simulink library "csu_esf_est_switch_frame_mtv_lib"  (R2014b)
settings: Solver=ode45  StartTime=0.0  StopTime=10.0  RelTol=1e-3
values from neighbouring files (symbols this model uses):
  kfl_accel_init = [0 0 0]'    [csc_kfl_kalman_filter_mtv_init.m]
  kfl_convergence_init = 2    [csc_kfl_kalman_filter_mtv_init.m]
  kfl_integrating_init = 1    [csc_kfl_kalman_filter_mtv_init.m]
  kfl_landed_init = 0    [csc_kfl_kalman_filter_mtv_init.m]
  kfl_quat_init = kfl_ic.quat_eci_to_body    [csc_est_state_estimation_test.m]    (also in csc_kfl_kalman_filter_mtv_init.m = [0 0 0 1]')
  kfl_rate_init = [ 0 0 0]'    [csc_kfl_kalman_filter_mtv_init.m]
  kfl_state_init = [ kfl_position_init ; kfl_velocity_init ; kfl_acc_bias_init ;  kfl_gibbs_init ;  kfl_gyro_bias_init]    [csc_est_state_estimation_test.m]
undefined symbols (not defined in the file or in its folder): ekf_covariance_init, elk_body_base_to_origin, elk_launchstand_height
libraries: simulink x2, util_info_lib x1, util_event_lib x1, util_fsw_frame_rotation_lib x1
settings Model: Creator=escrane  LastModifiedBy=mstewart

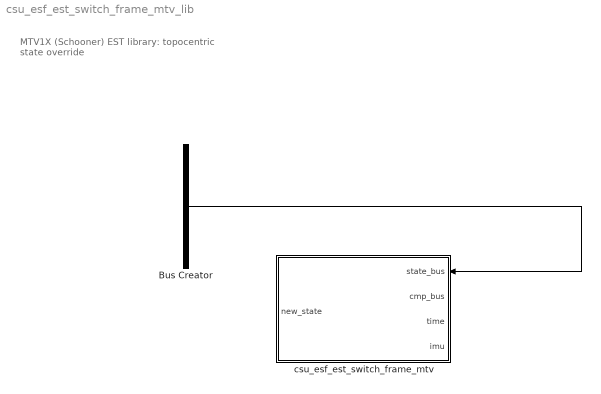
== system csu_esf_est_switch_frame_mtv_lib ==
  note: MTV1X (Schooner) EST library:
      | topocentric state override
  Bus Creator : BusCreator  Inputs=5
  csu_esf_est_switch_frame_mtv : Subsystem
  wires:
  Bus Creator/1 -> csu_esf_est_switch_frame_mtv/1(state_bus)
  ? -> Bus Creator/1  "x"
  ? -> Bus Creator/2  "accel"
  ? -> Bus Creator/3  "rate"
  ? -> Bus Creator/4  "q"
  ? -> Bus Creator/5  "P"

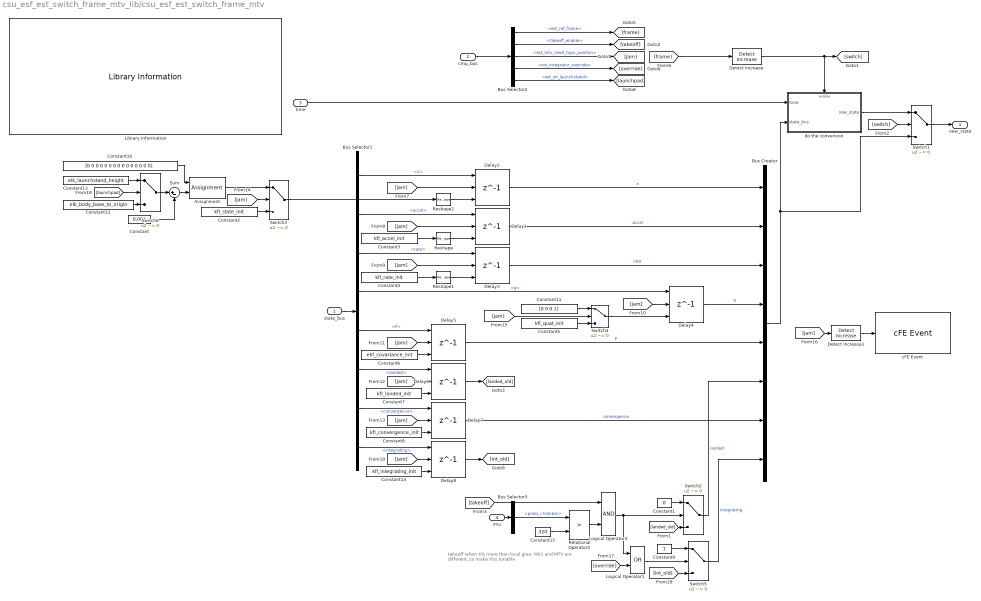
== system csu_esf_est_switch_frame_mtv_lib/csu_esf_est_switch_frame_mtv ==
  note: takeoff when X% more than local grav:
      | MX1 and MTV are different, so make this tunable
  state_bus : Inport
  cmp_bus : Inport  Port=2
  time : Inport  Port=3
  imu : Inport  Port=4
  Assignment : Assignment  DiagnosticForDimensions=Warning  Indices=3
  Bus Creator : BusCreator  Inputs=8
  Bus Selector1 : BusSelector  OutputSignals=x,accel,rate,q,P,landed,convergence,integrating
  Bus Selector2 : BusSelector  OutputSignals=est_ref_frame,takeoff_enable,est_mtv_reset_topo_position,est_integrator_override,est_on_launchstand
  Bus Selector3 : BusSelector  OutputSignals=press_chamber
  Constant : Constant  Value=0.001
  Constant1 : Constant  Value=0
  Constant10 : Constant  Value=[0 0 0 0 0 0 0 0 0 0 0 0 0 0 0]
  Constant11 : Constant  Value=[0 0 0 1]
  Constant12 : Constant  Value=elk_body_base_to_origin  VectorParams1D=off
  Constant13 : Constant  Value=elk_launchstand_height  VectorParams1D=off
  Constant14 : Constant  Value=kfl_integrating_init
  Constant15 : Constant  Value=320
  Constant2 : Constant  Value=kfl_state_init
  Constant3 : Constant  Value=kfl_accel_init
  Constant4 : Constant  Value=kfl_rate_init
  Constant5 : Constant  Value=kfl_quat_init
  Constant6 : Constant  Value=ekf_covariance_init
  Constant7 : Constant  Value=kfl_landed_init
  Constant8 : Constant  Value=kfl_convergence_init
  Constant9 : Constant
  Delay{1..8} (8 alike) : Delay  DelayLength=1  InitialConditionSource=Input port  ExternalReset=Rising
      settings: InputPortMap=u0,r5,p4
  Detect Increase : simulink/Logic and Bit Operations/Detect Increase  vinit=1  InputProcessing=Inherited  OutDataTypeStr=boolean
  Detect Increase1 : simulink/Logic and Bit Operations/Detect Increase  vinit=0  InputProcessing=Inherited  OutDataTypeStr=boolean
  Library Information : util_info_lib/Library Information  owner='escrane'
  Logical Operator1 : Logic  Operator=OR  AllPortsSameDT=off  OutDataTypeStr=boolean
  Logical Operator3 : Logic  AllPortsSameDT=off  OutDataTypeStr=boolean
  Relational Operator2 : RelationalOperator  Operator=>  OutDataTypeStr=boolean
  Reshape : Reshape  OutputDimensionality=Column vector (2-D)
  Reshape1 : Reshape  OutputDimensionality=Column vector (2-D)
  Reshape2 : Reshape  OutputDimensionality=Column vector (2-D)
  Sum : Sum  Inputs=|+-
  Switch{1..6} (6 alike) : Switch  Criteria=u2 ~= 0  Threshold=0.5  InputSameDT=on
  cFE Event : util_event_lib/cFE Event  event_message='Estimated topocentric state has been zeroed'  event_id=22  event_severity=INFORMATION  event_use_enums=off  event_enum_types={}
  do the conversion : Subsystem
  new_state : Outport
  wires:
  Constant15/1 -> Relational Operator2/2
  Bus Selector3/1 -> Relational Operator2/1  "<press_chamber>"
  imu/1 -> Bus Selector3/1
  [override] -> Logical Operator1/2
  Logical Operator1/1 -> Switch5/2
  [int_old] -> Switch5/3
  Constant14/1 -> Delay8/3
  [jam] -> Delay8/2
  Delay8/1 -> [int_old]
  Bus Selector1/8 -> Delay8/1  "<integrating>"
  Constant9/1 -> Switch5/1
  Switch5/1 -> Bus Creator/8  "integrating"
  Constant/1 -> Sum/2
  Switch6/1 -> Sum/1
  Sum/1 -> Assignment/2
  Constant10/1 -> Assignment/1
  Constant12/1 -> Switch6/3
  Constant13/1 -> Switch6/1
  [launchpad] -> Switch6/2
  Assignment/1 -> Switch3/1
  Bus Selector2/5 -> [launchpad]  "<est_on_launchstand>"
  Bus Selector2/4 -> [override]  "<est_integrator_override>"
  Detect Increase1/1 -> cFE Event/1
  [jam] -> Detect Increase1/1
  Bus Selector2/3 -> [jam]  "<est_mtv_reset_topo_position>"
  Switch4/1 -> Delay4/3
  Constant5/1 -> Switch4/3
  Constant11/1 -> Switch4/1
  [jam] -> Switch4/2
  Constant2/1 -> Switch3/3
  [jam] -> Switch3/2
  Switch3/1 -> Reshape2/1
  Reshape2/1 -> Delay2/3
  Reshape1/1 -> Delay3/3
  Reshape/1 -> Delay1/3
  Constant8/1 -> Delay7/3
  Constant7/1 -> Delay6/3
  Constant6/1 -> Delay5/3
  Constant4/1 -> Reshape1/1
  [jam] -> Delay7/2
  [jam] -> Delay6/2
  [jam] -> Delay5/2
  [jam] -> Delay3/2
  [jam] -> Delay4/2
  Constant3/1 -> Reshape/1
  [jam] -> Delay1/2
  [jam] -> Delay2/2
  [frame] -> Detect Increase/1
  Delay7/1 -> Bus Creator/7  "convergence"
  Bus Selector1/7 -> Delay7/1  "<convergence>"
  [landed_old] -> Switch2/3
  Delay6/1 -> [landed_old]
  Bus Selector2/2 -> [takeoff]  "<takeoff_enable>"
  Constant1/1 -> Switch2/1
  Switch2/1 -> Bus Creator/6  "landed"
  Logical Operator3/1 -> Switch2/2, Logical Operator1/1
  [takeoff] -> Logical Operator3/1
  Relational Operator2/1 -> Logical Operator3/2
  Bus Selector1/6 -> Delay6/1  "<landed>"
  state_bus/1 -> Bus Selector1/1
  Delay2/1 -> Bus Creator/1  "x"
  Delay1/1 -> Bus Creator/2  "accel"
  Delay3/1 -> Bus Creator/3  "rate"
  Delay4/1 -> Bus Creator/4  "q"
  Delay5/1 -> Bus Creator/5  "P"
  Bus Selector2/1 -> [frame]  "<est_ref_frame>"
  Detect Increase/1 -> do the conversion/Enable, [switch]
  do the conversion/1(new_state) -> Switch1/1
  [switch] -> Switch1/2
  Bus Selector1/1 -> Delay2/1  "<x>"
  Bus Selector1/2 -> Delay1/1  "<accel>"
  Bus Selector1/3 -> Delay3/1  "<rate>"
  Bus Selector1/4 -> Delay4/1  "<q>"
  Bus Selector1/5 -> Delay5/1  "<P>"
  Bus Creator/1 -> Switch1/3, do the conversion/2(state_bus)
  cmp_bus/1 -> Bus Selector2/1
  time/1 -> do the conversion/1(time)
  Switch1/1 -> new_state/1

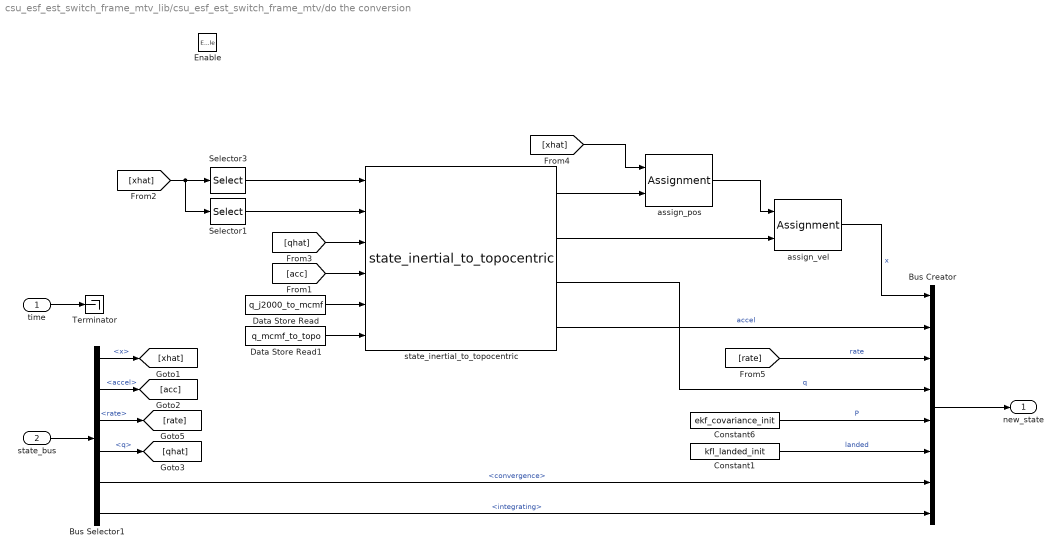
== system csu_esf_est_switch_frame_mtv_lib/csu_esf_est_switch_frame_mtv/do the conversion ==
  time : Inport
  state_bus : Inport  Port=2
  Enable : EnablePort
  Bus Creator : BusCreator  Inputs=8
  Bus Selector1 : BusSelector  OutputSignals=x,accel,rate,q,convergence,integrating
  Constant1 : Constant  Value=kfl_landed_init
  Constant6 : Constant  Value=ekf_covariance_init
  Data Store Read : DataStoreRead  DataStoreName=q_j2000_to_mcmf
  Data Store Read1 : DataStoreRead  DataStoreName=q_mcmf_to_topo
  Selector1 : Selector  InputPortWidth=kfl_n_state  Indices=kfl_vel_index
  Selector3 : Selector  InputPortWidth=kfl_n_state  Indices=kfl_pos_index
  Terminator : Terminator
  assign_pos : Assignment  Indices=kfl_pos_index
  assign_vel : Assignment  Indices=kfl_vel_index
  state_inertial_to_topocentric : util_fsw_frame_rotation_lib/state_inertial_to_topocentric  SystemSampleTime=-1
  new_state : Outport
  wires:
  Bus Selector1/6 -> Bus Creator/8  "<integrating>"
  time/1 -> Terminator/1
  Data Store Read/1 -> state_inertial_to_topocentric/5
  Data Store Read1/1 -> state_inertial_to_topocentric/6
  Bus Selector1/5 -> Bus Creator/7  "<convergence>"
  Constant1/1 -> Bus Creator/6  "landed"
  state_bus/1 -> Bus Selector1/1
  Bus Selector1/1 -> [xhat]  "<x>"
  Bus Selector1/2 -> [acc]  "<accel>"
  Bus Selector1/3 -> [rate]  "<rate>"
  Bus Selector1/4 -> [qhat]  "<q>"
  Bus Creator/1 -> new_state/1
  [rate] -> Bus Creator/3  "rate"
  [acc] -> state_inertial_to_topocentric/4
  [qhat] -> state_inertial_to_topocentric/3
  Constant6/1 -> Bus Creator/5  "P"
  state_inertial_to_topocentric/4 -> Bus Creator/2  "accel"
  state_inertial_to_topocentric/3 -> Bus Creator/4  "q"
  [xhat] -> Selector1/1, Selector3/1
  Selector3/1 -> state_inertial_to_topocentric/1
  Selector1/1 -> state_inertial_to_topocentric/2
  [xhat] -> assign_pos/1
  state_inertial_to_topocentric/1 -> assign_pos/2
  state_inertial_to_topocentric/2 -> assign_vel/2
  assign_pos/1 -> assign_vel/1
  assign_vel/1 -> Bus Creator/1  "x"
